simulink model "rtwdemo_parabuild_b_1"  (R2022b)
settings: Solver=FixedStepDiscrete  StartTime=0.0  StopTime=10.0  FixedStep=Auto  RelTol=1e-3  SampleTimeConstraint=STIndependent  EnableMultiTasking=on
Description:
  | Example model reference component.
settings Model: ModifiedByFormat=The MathWorks Inc.  Creator=The MathWorks, Inc.  LastModifiedBy=The MathWorks Inc.
settings SolverCC: AlgebraicLoopSolver=TrustRegion
settings DataIOCC: SaveFormat=StructureWithTime  SaveOutput=off  SaveTime=off  ReturnWorkspaceOutputs=off  SignalLoggingName=logsOut
settings OptimizationCC: DefaultParameterBehavior=Inlined  InlineInvariantSignals=on  EnhancedBackFolding=on  PassReuseOutputArgsAs=Individual arguments  ExpressionDepthLimit=2147483647  ZeroExternalMemoryAtStartup=off  ZeroInternalMemoryAtStartup=off  EfficientFloat2IntCast=on  EfficientMapNaN2IntZero=off  OptimizeBlockOrder=speed  DifferentSizesBufferReuse=on  OptimizationCustomize=off  EfficientTunableParamExpr=on
settings DebuggingCC: MergeDetectMultiDrivingBlocksExec=none  CheckExecutionContextPreStartOutputMsg=on  ParameterTunabilityLossMsg=error  FcnCallInpInsideContextMsg=warning  UnconnectedInputMsg=warning  UnconnectedOutputMsg=warning  UnconnectedLineMsg=warning  StateNameClashWarn=warning  StrictBusMsg=ErrorOnBusTreatedAsVector  SFUnexpectedBacktrackingDiag=warning  SFNoUnconditionalDefaultTransitionDiag=warning  SFExecutionAtInitializationDiag=none  SFMachineParentedDataDiag=warning  ArithmeticOperatorsInVariantConditions=warning
settings HardwareCC: TargetHWDeviceType=Generic->32-bit Embedded Processor
settings ModelReferenceCC: EnableRefExpFcnMdlSchedulingChecks=on  CheckModelReferenceTargetMessage=none  ModelReferencePassRootInputsByReference=off  PropagateSignalLabelsOutOfModel=off
settings SFSimCC: SimUseLocalCustomCode=off  MATLABDynamicMemAlloc=off  CustomCodeUndefinedFunction=UseInterfaceOnly
settings RTWCC: Description=Embedded Coder  SystemTargetFile=ert.tlc  TLCOptions=-p0 -aWarnNonSaturatedBlocks=0  TemplateMakefile=ert_default_tmf  GenerateReport=on  RTWVerbose=off  RTWUseLocalCustomCode=off  Toolchain=LCC-win64 v2.4.1 | gmake (64-bit Windows)  LaunchReport=on
settings CodeAppCC: ForceParamTrailComments=on  IgnoreCustomStorageClasses=off  MaxIdLength=128  OperatorAnnotations=on  SimulinkDataObjDesc=on  SFDataObjDesc=on  InsertBlockDesc=on
settings ERTTargetCC: GenerateSampleERTMain=on  InlinedParameterPlacement=NonHierarchical  ERTCustomFileTemplate=example_file_process.tlc
settings ConfigComp: CovMetricSettings=dw  CovSaveCumulativeToWorkspaceVar=on  CovSaveSingleToWorkspaceVar=on  CovExternalEMLEnable=off  CovSFcnEnable=off

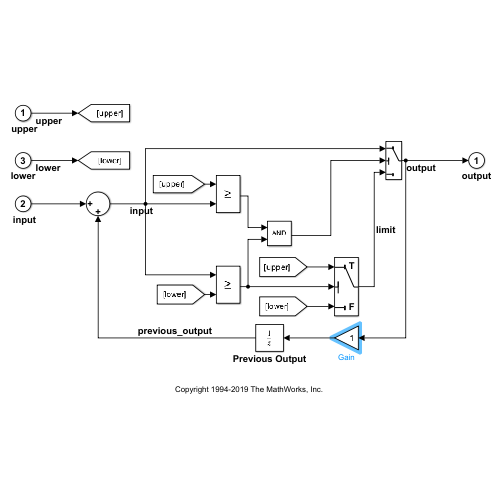
[thumbnail: Simulink's stored preview of the top-level diagram]
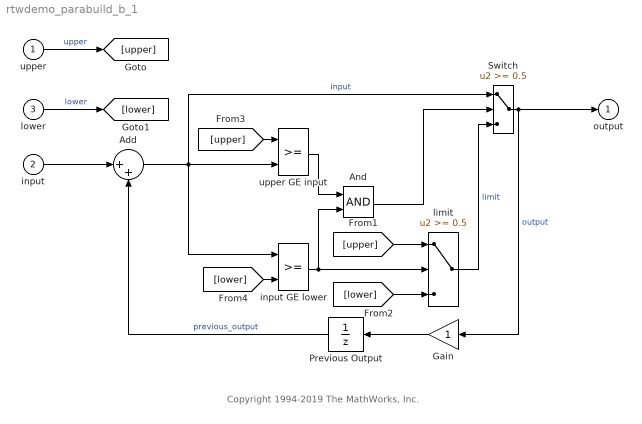
== system rtwdemo_parabuild_b_1 ==
  note: Copyright 1994-2019 The MathWorks, Inc.
  " upper" : Inport  OutDataTypeStr=double  PortDimensions=1
  " input" : Inport  Port=2  OutDataTypeStr=double  PortDimensions=1
  lower : Inport  Port=3  OutDataTypeStr=double  PortDimensions=1
  " input GE lower" : RelationalOperator  Priority=1  OutDataTypeStr=boolean
      settings: AttributesFormatString=\n
  " limit" : Switch  Threshold=0.5
  Add : Sum  Inputs=|++
  And : Logic  OutDataTypeStr=boolean
  Gain : Gain
  Previous Output : UnitDelay  SampleTime=-1  HasFrameUpgradeWarning=on
  Switch : Switch  Threshold=0.5
  upper GE input : RelationalOperator  Priority=0  OutDataTypeStr=boolean
      settings: AttributesFormatString=\n
  output : Outport  VectorParamsAs1DForOutWhenUnconnected=off
  wires:
  [upper] -> " limit"/1
  Switch/1 -> Gain/1, output/1  "output"
  " limit"/1 -> Switch/3  "limit"
  upper GE input/1 -> And/1
  Previous Output/1 -> Add/2  "previous_output"
  " input"/1 -> Add/1
  " upper"/1 -> [upper]  "upper"
  [lower] -> " limit"/3
  [upper] -> upper GE input/1
  [lower] -> " input GE lower"/2
  " input GE lower"/1 -> And/2, " limit"/2
  lower/1 -> [lower]  "lower"
  And/1 -> Switch/2
  Add/1 -> upper GE input/2, " input GE lower"/1, Switch/1  "input"
  Gain/1 -> Previous Output/1
